simulink model "demoWaypointGuidance"  (R2021a)
settings: Solver=ode45  StartTime=0.0  StopTime=50  MaxStep=10^-2  RelTol=1e-3  EnableMultiTasking=on
libraries: simulink x3, mssSimulink x1
settings Model: Creator=thor  LastModifiedBy=thor
settings SolverCC: AlgebraicLoopSolver=TrustRegion
settings DataIOCC: LimitDataPoints=on  SaveFormat=Array  SignalLoggingSaveFormat=ModelDataLogs  ReturnWorkspaceOutputs=off  SignalLoggingName=sigsOut
settings OptimizationCC: BooleanDataType=off  InitFltsAndDblsToZero=on  LifeSpan=inf
settings DebuggingCC: SaveWithParameterizedLinksMsg=none  UnderspecifiedInitializationDetection=Classic  MergeDetectMultiDrivingBlocksExec=none  SignalResolutionControl=TryResolveAllWithWarning  MultiTaskDSMMsg=warning  MultiTaskCondExecSysMsg=none  FcnCallInpInsideContextMsg=warning  SFUnexpectedBacktrackingDiag=warning  SFNoUnconditionalDefaultTransitionDiag=warning  SFExecutionAtInitializationDiag=none  SFMachineParentedDataDiag=warning  ArithmeticOperatorsInVariantConditions=warning
settings HardwareCC: ProdBitPerPointer=32  ProdBitPerSizeT=32  ProdBitPerPtrDiffT=32  ProdLargestAtomicFloat=None  ProdIntDivRoundTo=Undefined  ProdEndianess=Unspecified  ProdWordSize=32  ProdHWDeviceType=32-bit Generic  TargetUnknown=on
settings ModelReferenceCC: PropagateSignalLabelsOutOfModel=off
settings CodeAppCC: StateflowObjectComments=on
settings GRTTargetCC: TargetFcnLib=ansi_tfl_tmw.mat  TargetLangStandard=C89/C90 (ANSI)  ModelReferenceCompliant=off  ParMdlRefBuildCompliant=off  CompOptLevelCompliant=off  ConcurrentExecutionCompliant=off  CombineOutputUpdateFcns=off  MatFileLogging=off  MATLABClassNameForMDSCustomization=Simulink.SoftwareTarget.TargetSpecificTriggerConfigurationBase  GRTInterface=on
settings ConfigComp: CovMetricSettings=dw  CovSaveCumulativeToWorkspaceVar=on  CovSaveSingleToWorkspaceVar=on

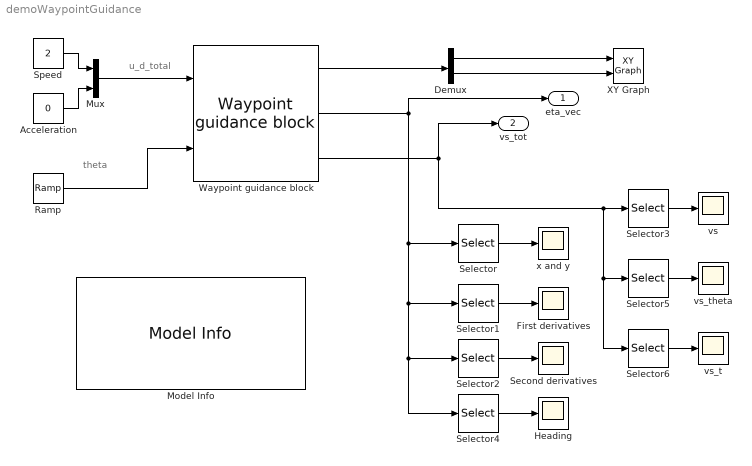
== system demoWaypointGuidance ==
  note: u_d_total
  note: theta
  Acceleration : Constant  Value=0
  Demux : Demux  Outputs=2
      settings: DisplayOption=none
  First derivatives : Scope
  Heading : Scope
  Model Info : simulink/Model-Wide Utilities/Model Info  Frame=on  DisplayStringWithTags=|  HorizontalTextAlignment=Left  LeftAlignmentValue=0.02
      | Waypoint guidance demo.
      | Creates a 3 times differentiable path between 
      | the provided waypoints. The user can choose
      | between cubic splines (3rd order)  and a 5th
      | order polynomial.
      | Author: Jørgen Corneliussen
      | %<ModifiedDate>
  Mux : Mux  Inputs=2
  "Ramp " : simulink/Sources/Ramp  slope=1  start=0  InitialOutput=0
  Second derivatives : Scope
  Selector : Selector  InputPortWidth=9  IndexOptions=Index vector (dialog)  Indices=[1 2]  OutputSizes=1
  Selector1 : Selector  InputPortWidth=9  IndexOptions=Index vector (dialog)  Indices=[4 5]  OutputSizes=1
  Selector2 : Selector  InputPortWidth=9  IndexOptions=Index vector (dialog)  Indices=[7 8]  OutputSizes=1
  Selector3 : Selector  InputPortWidth=3  IndexOptions=Index vector (dialog)  Indices=1  OutputSizes=1
  Selector4 : Selector  InputPortWidth=9  IndexOptions=Index vector (dialog)  Indices=3  OutputSizes=1
  Selector5 : Selector  InputPortWidth=3  IndexOptions=Index vector (dialog)  Indices=2  OutputSizes=1
  Selector6 : Selector  InputPortWidth=3  IndexOptions=Index vector (dialog)  Indices=3  OutputSizes=1
  Speed : Constant  Value=2
  "Waypoint guidance block " : mssSimulink/Guidance/Waypoint guidance block  x_vector=[-800 -500 -200 -50 -200 -250 200 500 500 300 0 -300 -600]  y_vector=[100 1800 2000 1500 1000 100 1000 300 -250 -200 100 -600 -1000]  method=5th order polynomial  drawmode=on  stop=on  mode=Acc  start=[100 0]  final=[0 100]  constraint=off
  XY Graph : simulink/Sinks/XY Graph  xmin=-800  xmax=600  ymin=-1500  ymax=2500  st=-1
  vs : Scope
  vs_t : Scope
  vs_theta : Scope
  x and y : Scope
  eta_vec : Outport
  vs_tot : Outport  Port=2
  wires:
  Speed/1 -> Mux/1
  Acceleration/1 -> Mux/2
  Mux/1 -> "Waypoint guidance block "/1
  "Waypoint guidance block "/2 -> Selector/1, Selector1/1, Selector2/1, Selector4/1, eta_vec/1
  "Ramp "/1 -> "Waypoint guidance block "/2
  "Waypoint guidance block "/3 -> Selector3/1, Selector6/1, Selector5/1, vs_tot/1
  Selector/1 -> x and y/1
  Selector1/1 -> First derivatives/1
  Selector2/1 -> Second derivatives/1
  "Waypoint guidance block "/1 -> Demux/1
  Selector3/1 -> vs/1
  Selector4/1 -> Heading/1
  Selector5/1 -> vs_theta/1
  Selector6/1 -> vs_t/1
  Demux/1 -> XY Graph/1
  Demux/2 -> XY Graph/2
